simulink library "lib_dynamic_saturator"  (R2023a)
settings: Solver=VariableStepAuto  StartTime=0.0  StopTime=10.0  RelTol=1e-3
settings Model: Creator=cav2ofo  LastModifiedBy=lenovo
settings OptimizationCC: ReuseModelBlockBuffer=off

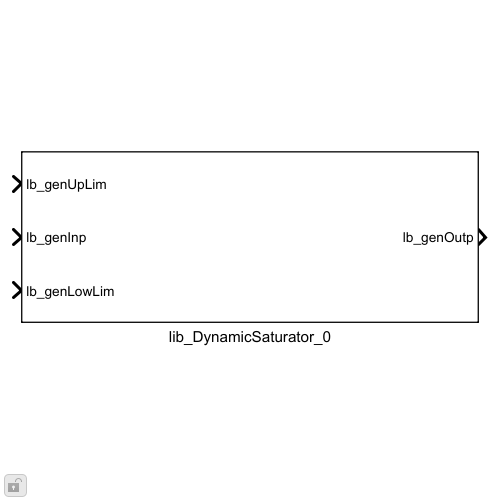
[thumbnail: Simulink's stored preview of the top-level diagram]
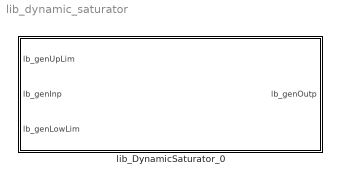
== system lib_dynamic_saturator ==
  lib_DynamicSaturator_0 : Subsystem
      mask DialogControl DescGroupVar Prompt: VHIT control library
      mask DialogControl DescTextVar Prompt: Dynamic saturator

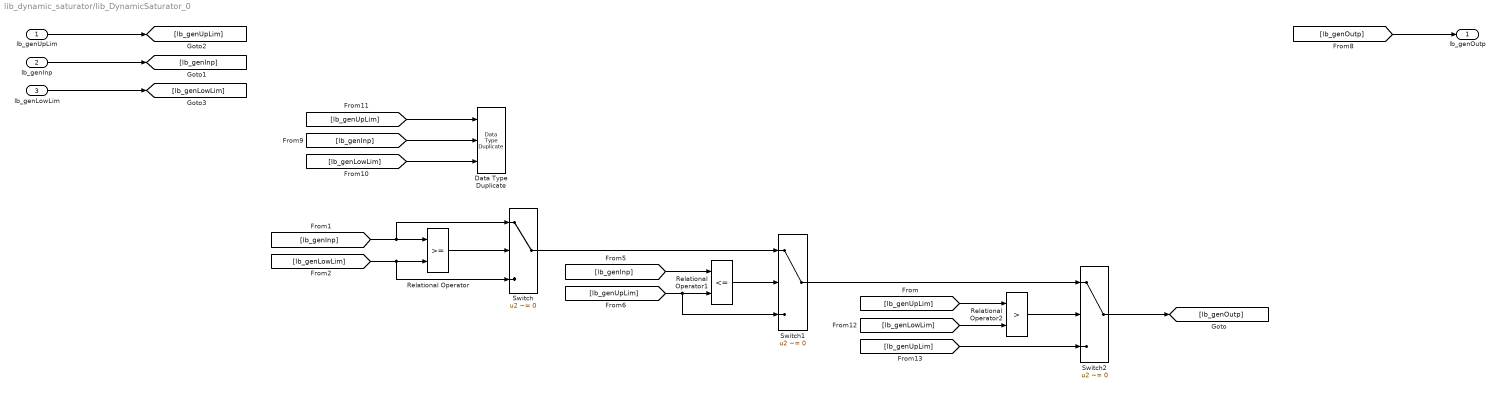
== system lib_dynamic_saturator/lib_DynamicSaturator_0 ==
  lb_genUpLim : Inport
  lb_genInp : Inport  Port=2
  lb_genLowLim : Inport  Port=3
  Data Type Duplicate : DataTypeDuplicate  NumInputPorts=3
  Relational Operator : RelationalOperator  OutDataTypeStr=boolean  RndMeth=Simplest  InputSameDT=off
  Relational Operator1 : RelationalOperator  Operator=<=  OutDataTypeStr=boolean  RndMeth=Simplest  InputSameDT=off
  Relational Operator2 : RelationalOperator  Operator=>  OutDataTypeStr=boolean  RndMeth=Simplest  InputSameDT=off
  Switch : Switch  Criteria=u2 ~= 0  SaturateOnIntegerOverflow=off  InputSameDT=off
  Switch1 : Switch  Criteria=u2 ~= 0  SaturateOnIntegerOverflow=off  InputSameDT=off
  Switch2 : Switch  Criteria=u2 ~= 0  SaturateOnIntegerOverflow=off  InputSameDT=off
  lb_genOutp : Outport
  wires:
  lb_genUpLim/1 -> [lb_genUpLim]
  lb_genInp/1 -> [lb_genInp]
  lb_genLowLim/1 -> [lb_genLowLim]
  [lb_genInp] -> Switch/1, Relational Operator/1
  [lb_genLowLim] -> Relational Operator/2, Switch/3
  Relational Operator/1 -> Switch/2
  Relational Operator1/1 -> Switch1/2
  [lb_genOutp] -> lb_genOutp/1
  [lb_genUpLim] -> Data Type Duplicate/1
  [lb_genInp] -> Data Type Duplicate/2
  [lb_genLowLim] -> Data Type Duplicate/3
  [lb_genLowLim] -> Relational Operator2/2
  [lb_genUpLim] -> Relational Operator2/1
  Relational Operator2/1 -> Switch2/2
  Switch1/1 -> Switch2/1
  [lb_genUpLim] -> Switch2/3
  Switch2/1 -> [lb_genOutp]
  [lb_genInp] -> Relational Operator1/1
  [lb_genUpLim] -> Switch1/3, Relational Operator1/2
  Switch/1 -> Switch1/1
